simulink model "plot_robot"  (R2022b)
settings: Solver=VariableStepAuto  StartTime=0.0  StopTime=10.0  RelTol=1e-3
settings Model: Creator=User  LastModifiedBy=User

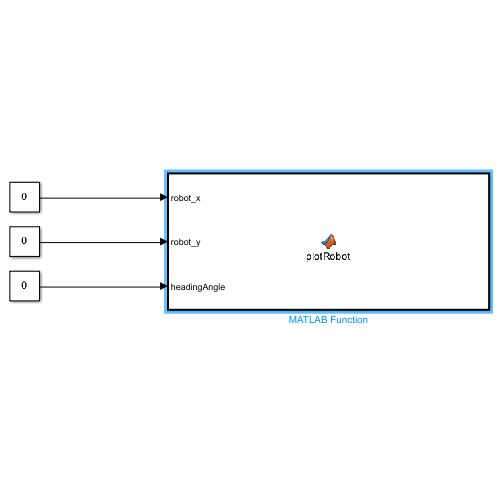
[thumbnail: Simulink's stored preview of the top-level diagram]
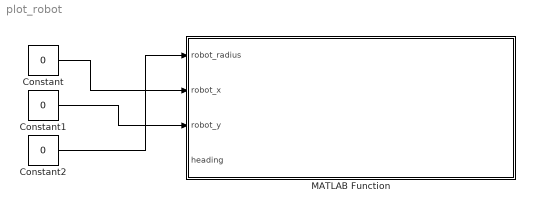
== system plot_robot ==
  Constant : Constant  Value=0
  Constant1 : Constant  Value=0
  Constant2 : Constant  Value=0
  MATLAB Function : MATLAB Function  InitFcn=|  TreatAsAtomicUnit=on
      | figure(1); clf; hold on; grid on; axis([-45,45,-30,30]);
      | p = plot(30,20,'Marker','+','Color','b');
  wires:
  Constant2/1 -> MATLAB Function/1(robot_radius)
  Constant1/1 -> MATLAB Function/3(robot_y)
  Constant/1 -> MATLAB Function/2(robot_x)

== matlab function plot_robot/MATLAB Function ==
  data: robot_radius input; robot_x input; robot_y input; heading input
function plotRobot(robot_radius, robot_x, robot_y, heading)

    theta    = linspace(0, 2*pi, 360);   
    
    robot_rep_x = robot_radius * cos(theta);
    robot_rep_y = robot_radius * sin(theta);

    heading_line_x = cos(heading) * (robot_radius + 4);
    heading_line_y = sin(heading) * (robot_radius + 4);

    % Draw circle around current location of robot
    p = plot((robot_rep_x + robot_x), (robot_rep_y + robot_y), 'b');
    
    % Draw line from center of robot in the direction of the current heading
    line([robot_x, (heading_line_y + robot_x)], [robot_y, (heading_line_x + robot_y)], 'color', 'b');

    drawnow();

end
